simulink model "MicrogridDynamics"  (R2020b)
settings: Solver=ode23t  StartTime=0.0  StopTime=1  RelTol=1e-3
values from neighbouring files (symbols this model uses):
  C = 10e-6    (= 1e-05)    [ControllerDesign.m]
  Frq = 50    [ControllerDesign.m]
  Lg = 1.5e-3    (= 0.0015)    [ControllerDesign.m]
  Li = 3e-3    (= 0.003)    [ControllerDesign.m]
  Ll = 10e-3    (= 0.01)    [ControllerDesign.m]
  Rl = 1    [ControllerDesign.m]
  Rld = 50    [ControllerDesign.m]
  Rld1 = 200    [ControllerDesign.m]
  sw_fr = 10e3    (= 10000)    [ControllerDesign.m]
  Vac = 220    [ControllerDesign.m]
  Vdc = 500    [ControllerDesign.m]
undefined symbols (not defined in the file or in its folder): C_pi, C_pi1
libraries: powerlib x61, powerlib_meascontrol x12, pid_lib x8, eeRmsMeasurement x4, eePowerMeasurement x2
(part 2 of 2)

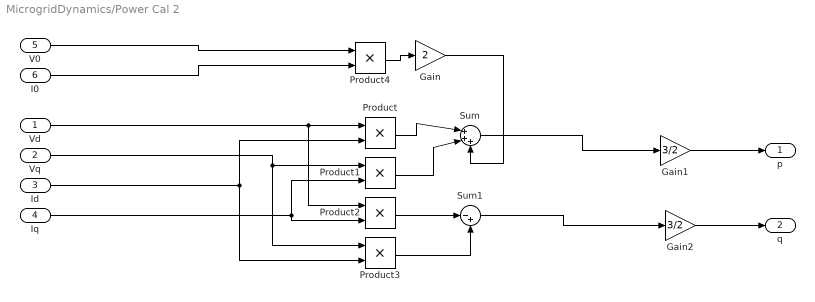
== system MicrogridDynamics/Power Cal 2 ==
  Vd : Inport
  Vq : Inport  Port=2
  Id : Inport  Port=3
  Iq : Inport  Port=4
  V0 : Inport  Port=5
  I0 : Inport  Port=6
  Gain : Gain  Gain=2
  Gain1 : Gain  Gain=3/2
  Gain2 : Gain  Gain=3/2
  Product{,1..4} (5 alike) : Product
  Sum : Sum  Inputs=|+++
  Sum1 : Sum  Inputs=|-+
  p : Outport
  q : Outport  Port=2
  wires:
  Sum1/1 -> Gain2/1
  Product/1 -> Sum/1
  Id/1 -> Product/2, Product3/2
  Product1/1 -> Sum/2
  Product2/1 -> Sum1/1
  Vd/1 -> Product2/1, Product/1
  Sum/1 -> Gain1/1
  Product3/1 -> Sum1/2
  Vq/1 -> Product3/1, Product1/1
  Iq/1 -> Product1/2, Product2/2
  V0/1 -> Product4/1
  I0/1 -> Product4/2
  Product4/1 -> Gain/1
  Gain/1 -> Sum/3
  Gain1/1 -> p/1
  Gain2/1 -> q/1

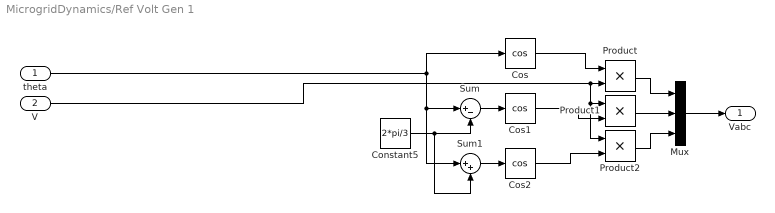
== system MicrogridDynamics/Ref Volt Gen 1 ==
  theta : Inport
  V : Inport  Port=2
  Constant5 : Constant  Value=2*pi/3
  Cos : Trigonometry  Operator=cos
  Cos1 : Trigonometry  Operator=cos
  Cos2 : Trigonometry  Operator=cos
  Mux : Mux  Inputs=3
  Product : Product
  Product1 : Product
  Product2 : Product
  Sum : Sum  Inputs=|+-
  Sum1 : Sum  Inputs=|++
  Vabc : Outport
  wires:
  Sum/1 -> Cos1/1
  Constant5/1 -> Sum1/2, Sum/2
  Mux/1 -> Vabc/1
  Sum1/1 -> Cos2/1
  Cos2/1 -> Product2/2
  Cos/1 -> Product/1
  Cos1/1 -> Product1/2
  Product2/1 -> Mux/3
  Product/1 -> Mux/1
  Product1/1 -> Mux/2
  V/1 -> Product/2, Product1/1, Product2/1
  theta/1 -> Cos/1, Sum/1, Sum1/1

== system MicrogridDynamics/Ref Volt Gen 2 ==
  theta : Inport
  V : Inport  Port=2
  Constant5 : Constant  Value=2*pi/3
  Cos : Trigonometry  Operator=cos
  Cos1 : Trigonometry  Operator=cos
  Cos2 : Trigonometry  Operator=cos
  Mux : Mux  Inputs=3
  Product : Product
  Product1 : Product
  Product2 : Product
  Sum : Sum  Inputs=|+-
  Sum1 : Sum  Inputs=|++
  Vabc : Outport
  wires:
  Sum/1 -> Cos1/1
  Constant5/1 -> Sum1/2, Sum/2
  Mux/1 -> Vabc/1
  Sum1/1 -> Cos2/1
  Cos2/1 -> Product2/2
  Cos/1 -> Product/1
  Cos1/1 -> Product1/2
  Product2/1 -> Mux/3
  Product/1 -> Mux/1
  Product1/1 -> Mux/2
  V/1 -> Product/2, Product1/1, Product2/1
  theta/1 -> Cos/1, Sum/1, Sum1/1

== system MicrogridDynamics/Scope ==
  "AC Grid Reference RMS Voltage  " : Inport
  "Inverter-1 RMS Voltage  " : Inport  Port=2
  Inverter-1 Voltage Profile : Inport  Port=3
  Inverter-2 Voltage Profile : Inport  Port=4
  Load Current Profile : Inport  Port=5
  Scope : Scope
  Scope2 : Scope
  Scope8 : Scope
  Voltage Profile : Scope  NumInputPorts=2
  wires:
  Inverter-1 Voltage Profile/1 -> Scope/1
  "AC Grid Reference RMS Voltage  "/1 -> Voltage Profile/1
  Inverter-2 Voltage Profile/1 -> Scope2/1
  "Inverter-1 RMS Voltage  "/1 -> Voltage Profile/2
  Load Current Profile/1 -> Scope8/1

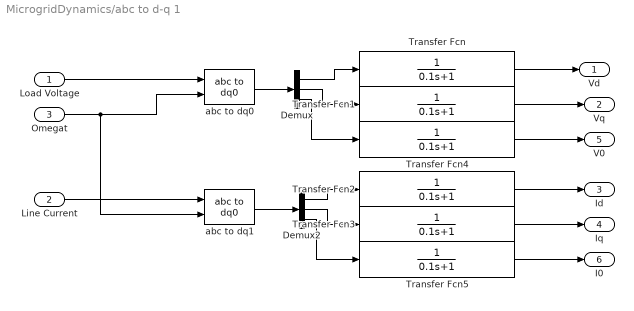
== system MicrogridDynamics/abc to d-q 1 ==
  Load Voltage : Inport
  Line Current : Inport  Port=2
  Omegat : Inport  Port=3
  Demux : Demux  Outputs=3
  Demux2 : Demux  Outputs=3
  Transfer Fcn{,1..5} (6 alike) : TransferFcn  Denominator=[0.1 1]
  abc to dq0 : powerlib_meascontrol/Transformations/abc to dq0  Alignment=90 degrees behind phase A axis
  abc to dq1 : powerlib_meascontrol/Transformations/abc to dq0  Alignment=90 degrees behind phase A axis
  Vd : Outport
  Vq : Outport  Port=2
  Id : Outport  Port=3
  Iq : Outport  Port=4
  V0 : Outport  Port=5
  I0 : Outport  Port=6
  wires:
  Load Voltage/1 -> abc to dq0/1
  abc to dq1/1 -> Demux2/1
  Omegat/1 -> abc to dq1/2, abc to dq0/2
  abc to dq0/1 -> Demux/1
  Line Current/1 -> abc to dq1/1
  Demux/1 -> Transfer Fcn/1
  Demux/2 -> Transfer Fcn1/1
  Demux2/1 -> Transfer Fcn2/1
  Demux2/2 -> Transfer Fcn3/1
  Transfer Fcn/1 -> Vd/1
  Transfer Fcn1/1 -> Vq/1
  Transfer Fcn2/1 -> Id/1
  Transfer Fcn3/1 -> Iq/1
  Demux/3 -> Transfer Fcn4/1
  Transfer Fcn4/1 -> V0/1
  Demux2/3 -> Transfer Fcn5/1
  Transfer Fcn5/1 -> I0/1

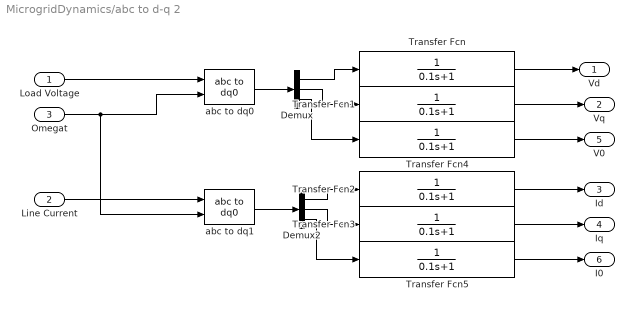
== system MicrogridDynamics/abc to d-q 2 ==
  Load Voltage : Inport
  Line Current : Inport  Port=2
  Omegat : Inport  Port=3
  Demux : Demux  Outputs=3
  Demux2 : Demux  Outputs=3
  Transfer Fcn{,1..5} (6 alike) : TransferFcn  Denominator=[0.1 1]
  abc to dq0 : powerlib_meascontrol/Transformations/abc to dq0  Alignment=90 degrees behind phase A axis
  abc to dq1 : powerlib_meascontrol/Transformations/abc to dq0  Alignment=90 degrees behind phase A axis
  Vd : Outport
  Vq : Outport  Port=2
  Id : Outport  Port=3
  Iq : Outport  Port=4
  V0 : Outport  Port=5
  I0 : Outport  Port=6
  wires:
  Load Voltage/1 -> abc to dq0/1
  abc to dq1/1 -> Demux2/1
  Omegat/1 -> abc to dq1/2, abc to dq0/2
  abc to dq0/1 -> Demux/1
  Line Current/1 -> abc to dq1/1
  Demux/1 -> Transfer Fcn/1
  Demux/2 -> Transfer Fcn1/1
  Demux2/1 -> Transfer Fcn2/1
  Demux2/2 -> Transfer Fcn3/1
  Transfer Fcn/1 -> Vd/1
  Transfer Fcn1/1 -> Vq/1
  Transfer Fcn2/1 -> Id/1
  Transfer Fcn3/1 -> Iq/1
  Demux/3 -> Transfer Fcn4/1
  Transfer Fcn4/1 -> V0/1
  Demux2/3 -> Transfer Fcn5/1
  Transfer Fcn5/1 -> I0/1
